simulink model "bus_roadtest_v3"  (R2018a)
settings: Solver=ode3  StartTime=0.0  StopTime=inf  FixedStep=0.01  RelTol=1e-3  EnableMultiTasking=on
PostLoadFcn:
  | , if any(exist('dsrtsu_mdlpostloadfcn', 'file') == [2, 3, 6]), try dsrtsu_mdlpostloadfcn('Execute', bdroot); catch fprintf('Error in PostLoadFcn (dsrtsu_mdlpostloadfcn) for model "%s":\n %s\n', bdroot, lasterr); end, end,
InitFcn:
  | bus_roadtest_v3_initial
values from neighbouring files (symbols this model uses):
  ay_max = 2    [Ini.m]
  delta_t = 0.01    [Ini.m]
  end_left_pass = 1    [Ini.m]
  end_right_pass = 0    [Ini.m]
  finish_node_id = length(Map_data(:,1))    [Ini.m]
  forward_length = 15    [Ini.m]
  gamma = sqrt(N_xaug+lambda)    [bus_roadtest_v3_initial.m]
  k_safe = 1    [Ini.m]
  nodes = nodes(1:index_node,:)    [Ini.m]
  rmin = 10    [Ini.m]
  segments = zeros(length(xy_ends_Pos(:,1)),3)    [Ini.m]
  start_node_id = 1    [Ini.m]
  Ts = 0.01    [bus_roadtest_v3_initial.m]
  Veh_CG = [0.5, 0.2]    [Ini.m]
  Veh_size = [1.99986,6.09558]    [Ini.m]
  vmax = 6    [Ini.m]
  weight = [weight_0,weight_0_cov,weight_i]    [bus_roadtest_v3_initial.m]
undefined symbols (not defined in the file or in its folder): Brake_table, DiscIntNeverNeededParam, Map_data, R, REF_GPS_RFS, Steer_gain_table, T
libraries: rtican x71, simulink x26, rti1401lib_adc_type4 x8, rti1401lib_dio_type4 x1
(part 1 of 18)
settings Model: DSRTSU_INTERNAL_RTI_VER=520  DSRTSU_INTERNAL_RTI_TYPE=rti1401  DSRTSU_INTERNAL_RTIFPGA=110  RTICANMMDATA=struct('GeneralSetupData',struct('modelroot','C:\Users\ITRI\Desktop\CarB_v3','generalsettings',struct('filesettings',struct('destfolder',struct('Name','RTICANMM_FILES','Check',1),'buildfolder',struct('Name','.','Check',1),'AbsDestfolder',struct('Name','C:\Users\ITRI\Desktop\CarB_v3\RTICANMM_FILES'),'AbsBuildfolder',struct('Name','C:\Users\ITRI\Desktop\CarB_v3'))),'options',struct('addpaths',1,'rmpaths',1,'addtrcexclusion',logical(1),'cannavigator',struct('checkmonitoring',0),'show_usrtrc',0,'use_usrtrc',0),'advanced',struct('options',[1 1 1 1 1 1 1 1 1 1 1 1 1 1 1 1 1 1 1 1 1 1 1 1 1 1 1 1 1 1 1 1 1 1 1 1 1 1 1 1 1 1 1 1 1 1 1 1 1 1 1 1 1 1 1 1 1 1 1 1 1 1 1 1 1 1 1 1 1 1 1 1 1 1 1 1 1 1 1 1 1 1 1 1 1 1 1 1 1 1 1 1 1 1 1 1 1 1 1 1]),'MPSetup',{{}},'modelname','bus_roadtest_v3','block','bus_roadtest_v3'))  DSRTSU_INTERNAL_RTIFLEXRAYCONFIG=110  Creator=LABTEST  LastModifiedBy=ITRI
settings DataIOCC: LimitDataPoints=on  SaveFormat=Array
settings OptimizationCC: BlockReduction=off  OptimizeBlockIOStorage=off  BufferReuse=off  GlobalBufferReuse=off  ExpressionFolding=off  ExpressionDepthLimit=2147483647  LocalBlockOutputs=off  LifeSpan=inf  OptimizeDataStoreBuffers=off  BusAssignmentInplaceUpdate=off
settings DebuggingCC: UnderspecifiedInitializationDetection=Classic  MergeDetectMultiDrivingBlocksExec=none  SolverPrmCheckMsg=warning  StateNameClashWarn=warning  SFUnexpectedBacktrackingDiag=warning  SFNoUnconditionalDefaultTransitionDiag=warning  SFExecutionAtInitializationDiag=none
settings HardwareCC: ProdBitPerPointer=32  ProdBitPerSizeT=32  ProdBitPerPtrDiffT=32  ProdLargestAtomicInteger=Integer  ProdEndianess=BigEndian  ProdWordSize=32  ProdHWDeviceType=Custom Processor->Custom  TargetIntDivRoundTo=Zero  TargetEndianess=BigEndian  TargetHWDeviceType=Custom Processor->Custom
settings ModelReferenceCC: PropagateSignalLabelsOutOfModel=off
settings SFSimCC: MATLABDynamicMemAlloc=off
settings RTWCC: SystemTargetFile=rti1401.tlc  MakeCommand=make_rti  TemplateMakefile=rti1401.tmf  Description=dSPACE DS1401 Hardware Platform
settings CodeAppCC: StateflowObjectComments=on
settings STFCustomTargetCC: ParMdlRefBuildCompliant=on  GRTInterface=off  SystemTargetFile=rti1401.tlc
settings GRTTargetCC: TargetLangStandard=C89/C90 (ANSI)  CompOptLevelCompliant=off  ConcurrentExecutionCompliant=off  CombineOutputUpdateFcns=off  MatFileLogging=off  CPPClassGenCompliant=off  UseToolchainInfoCompliant=off  ExtModeMexFile=noextcomm
settings ConfigComp: CovMetricSettings=dw  CovHtmlReporting=on  CovSaveCumulativeToWorkspaceVar=on  CovSaveSingleToWorkspaceVar=on  CovExternalEMLEnable=off
settings SimscapeCC: SimscapeNormalizeSystem=off
settings ConfigurationSet: Description=SimMechanics 2G

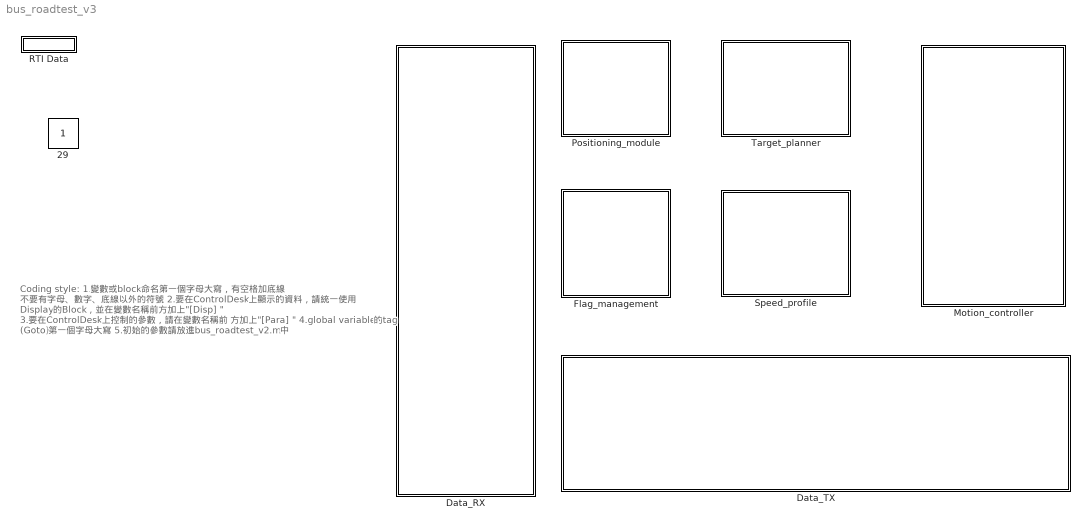
== system bus_roadtest_v3 ==
  note: Coding style:
      | 1.變數或block命名第一個字母大寫，有空格加底線
      | 不要有字母、數字、底線以外的符號
      | 2.要在ControlDesk上顯示的資料，請統一使用
      | Display的Block，並在變數名稱前方加上"[Disp] "
      | 3.要在ControlDesk上控制的參數，請在變數名稱前
      | 方加上"[Para] "
      | 4.global variable的tag (Goto)第一個字母大寫
      | 5.初始的參數請放進bus_roadtest_v2.m中
  Data_RX : Subsystem
  Data_TX : Subsystem
  Flag_management : Subsystem
  Motion_controller : Subsystem
  Positioning_module : Subsystem
  RTI Data : Subsystem  Tag=struct('RTIDataServer',struct('RTIDataServerVs','2','RTIModelDescription','struct(''main'',''bus_roadtest_v3'',''sub'','''',''isMp'',0)'))  LoadFcn="if exist('rtidc'), try,  rtidc('DataHostBlockClbLoad', gcbh); catch, disp(['Warning: ''LoadFcn'' for RTI Data block failed: ' lasterr]); end, end,"  mask(RTI_DATA_HOST){}
      mask help:
      | RTI Data Block.
      | This block is used by RTI to store internal model-dependent data.
      | Please keep this block on the root level of the model. Deleting this block will result in data loss.
      |
      | NEVER DELETE OR COPY THIS BLOCK!
      settings: CopyFcn="if exist('rtidc'), try,  rtidc('DataHostBlockClbCopy', gcbh); catch, disp(['Warning: ''CopyFcn'' for RTI Data block failed: ' lasterr]); end, end,"  DeleteFcn="if exist('rtidc'), try,  rtidc('DataHostBlockClbDelete', gcbh); catch, disp(['Warning: ''DeleteFcn'' for RTI Data block failed: ' lasterr]); end, end,"  ModelCloseFcn="if exist('rtidc'), try,  rtidc('DataHostBlockClbModelClose', gcbh); catch, disp(['Warning: ''ModelCloseFcn'' for RTI Data block failed: ' lasterr]); end, end,"  PreSaveFcn="if exist('rtidc'), try,  rtidc('DataHostBlockClbPreSave', gcbh); catch, disp(['Warning: ''PreSaveFcn'' for RTI Data block failed: ' lasterr]); end, end,"  PostSaveFcn="if exist('rtidc'), try,  rtidc('DataHostBlockClbPostSave', gcbh); catch, disp(['Warning: ''PostSaveFcn'' for RTI Data block failed: ' lasterr]); end, end,"  NameChangeFcn="if exist('rtidc'), try,  rtidc('DataHostBlockClbNameChange', gcbh); catch, disp(['Warning: ''NameChangeFcn'' for RTI Data block failed: ' lasterr]); end, end,"
      mask Help:
      | RTI Data Block.
      | This block is used by RTI to store internal model-dependent data.
      | Please keep this block on the root level of the model. Deleting this block will result in data loss.
      | 
      | NEVER DELETE OR COPY THIS BLOCK!
      mask Display:
      | text(0.5, 0.5, 'RTI Data', 'HorizontalAlignment', 'center');
      | plot([1 0]);
  Speed_profile : Subsystem
  Target_planner : Subsystem
  29 : Constant  IOType=siggen

== system bus_roadtest_v3/Data_RX ==
  note: 請把處理完的資料放在各自的Block裡面
      | 用global variable傳
  Control_button : Subsystem
  OBU : Subsystem
  PLC : Subsystem
  SBG : Subsystem
  X-by-wire : Subsystem
  Xavier : Subsystem

== system bus_roadtest_v3/Data_TX ==
  ARTC : Subsystem
  IPC : Subsystem

== system bus_roadtest_v3/Flag_management ==
  AEB_Enable : Constant
  AEB_Set : Constant  Value=0
  Button management : Subsystem
  Fault detection : Subsystem
  MATLAB Function : MATLAB Function  TreatAsAtomicUnit=on
  Memory : Memory
  Multiport Switch : MultiPortSwitch  DataPortOrder=Specify indices
  Multiport Switch1 : MultiPortSwitch  DataPortOrder=Specify indices
  OR : Logic  Operator=OR  IconShape=distinctive  AllPortsSameDT=off  OutDataTypeStr=boolean
  OR1 : Logic  Operator=OR  IconShape=distinctive  AllPortsSameDT=off  OutDataTypeStr=boolean
  Slow_flag : Constant  Value=0
  State management : Subsystem
  State toggle : MATLAB Function  TreatAsAtomicUnit=on
  "[Disp] AEB_flag_final" : Scope
  "[Disp] Drive_start" : Display
  "[Disp] Drive_state" : Display
  "[Disp] Drive_stop" : Display
  "[Disp] Self_driving_on" : Display
  "[Para] Button_on" : Constant
  "[Para] Door_cmd" : Constant  Value=0
  "[Para] Drive_start" : Constant  Value=0
  "[Para] Drive_stop" : Constant  Value=0
  "[Para] Emergency_stop" : Constant  Value=0
  "[Para] Fault_minor" : Constant  Value=0
  "[Para] Fault_prime" : Constant  Value=0
  switch : Switch  Criteria=u2 > Threshold
  tag scope: AEB_flag=global, BusStop_flag=global, Door_cmd=global, Drive_start=global, Drive_stop=global, Emergency_stop=global, Fault_minor=global, Fault_prime=global, Idle_flag=global, Light_flag=global, Obj_detect=global, Self_driving_on=global, Slow_flag=global, Stop_Check=global, Uturn_flag=global
  wires:
  State management/1(Idle_flag) -> [Idle_flag]
  State management/6(Obj_detect) -> [Obj_detect]
  State management/5(Stop_Check) -> [Stop_Check]
  State management/7(Light_flag) -> [Light_flag]
  State management/8(BusStop_flag) -> [BusStop_flag]
  "[Para] Door_cmd"/1 -> [Door_cmd]
  "[Para] Emergency_stop"/1 -> [Emergency_stop]
  switch/1 -> "[Disp] AEB_flag_final"/1, [AEB_flag]
  AEB_Enable/1 -> switch/2
  AEB_Set/1 -> switch/3
  State management/3(AEB_flag) -> switch/1
  Slow_flag/1 -> [Slow_flag]
  "[Para] Fault_minor"/1 -> [Fault_minor]
  "[Para] Fault_prime"/1 -> [Fault_prime]
  Multiport Switch/1 -> "[Disp] Drive_start"/1, [Drive_start], State toggle/1(Drive_start)
  "[Para] Drive_stop"/1 -> Multiport Switch1/2
  Multiport Switch1/1 -> "[Disp] Drive_stop"/1, State toggle/2(Drive_stop), [Drive_stop]
  "[Para] Button_on"/1 -> Multiport Switch/1, Multiport Switch1/1
  State management/4(Uturn_flag) -> [Uturn_flag]
  [Static_flag] -> State toggle/3(Static_flag)
  State toggle/1(Self_driving_on) -> Memory/1, "[Disp] Self_driving_on"/1, [Self_driving_on]
  "[Para] Drive_start"/1 -> Multiport Switch/2
  [TouchP_start] -> MATLAB Function/3(TouchP_start)
  MATLAB Function/1(Drive_start) -> OR/2
  [Drive_start_button] -> OR/1, Multiport Switch/3
  [Drive_stop_button] -> OR1/2, Multiport Switch1/3
  MATLAB Function/2(Drive_stop) -> OR1/1
  OR1/1 -> Multiport Switch1/4
  OR/1 -> Multiport Switch/4
  [System_ready] -> MATLAB Function/5(System_ready)
  Memory/1 -> MATLAB Function/6(Actual_state)
  [AEB_flag] -> State toggle/4(AEB_flag)
  [TouchP_start_RX] -> MATLAB Function/4(TouchP_start_RX)
  [Drive_start_button] -> MATLAB Function/1(Drive_start_button)
  [Drive_stop_button] -> MATLAB Function/2(Drive_stop_button)
  MATLAB Function/3(Drive_state_out) -> "[Disp] Drive_state"/1
  [Idle_flag] -> State toggle/5(Idle_flag)

== system bus_roadtest_v3/Motion_controller ==
  Auto_flag : Constant
  Constant : Constant  Value=0
  Lateral_control : Subsystem
  Longitudinal_control : Subsystem
  Speed_cmd : Constant  Value=0
  Switch : Switch  Criteria=u2 > Threshold
  Switch1 : Switch  Criteria=u2 > Threshold
  Switch2 : Switch  Criteria=u2 > Threshold
  "[Disp] Speed_cmd" : Display
  "[Para]Speed_cmd_switch" : Constant  Value=0
  wires:
  Switch/1 -> Longitudinal_control/1(Speed_profile), "[Disp] Speed_cmd"/1
  "[Para]Speed_cmd_switch"/1 -> Switch/2
  [Speed_cmd] -> Switch/1
  Speed_cmd/1 -> Switch/3
  Switch1/1 -> Longitudinal_control/2(AEB_trig)
  [AEB_flag] -> Switch1/1
  Constant/1 -> Switch2/3, Switch1/3
  Switch2/1 -> Longitudinal_control/3(Static)
  [Static_flag] -> Switch2/1
  Auto_flag/1 -> Switch2/2, Switch1/2

== system bus_roadtest_v3/Positioning_module ==
  note: 綠底部分為從感測器進來的資訊
  Constant2 : Constant  Value=REF_GPS_RFS
  Gain : Gain  Gain=pi/180
  ITRI_MM : Subsystem
  "[Disp] Sensor_Velocity" : Display
  "[Para] D_GC" : Constant  Value=3.8
  wires:
  [MB5000_Latitude] -> ITRI_MM/2(GPS_LAT)
  [MB5000_Longitude] -> ITRI_MM/1(GPS_LONG)
  [MB5000_Altitude] -> ITRI_MM/3(GPS_ALT)
  [SBG_Course] -> ITRI_MM/6(course)
  Constant2/1 -> ITRI_MM/7(REF_GPS_RFS)
  [SBG_GPS_TYPE] -> ITRI_MM/8(SBG_GPS_TYPE)
  [MB5000_X_Acc] -> ITRI_MM/9(GPS_X_ACC)
  [MB5000_Y_Acc] -> ITRI_MM/10(GPS_Y_ACC)
  [SBG_Longitude] -> ITRI_MM/11(SBG_long)
  [SBG_Latitude] -> ITRI_MM/12(SBG_lat)
  [SBG_Altitude] -> ITRI_MM/13(SBG_alt)
  [SBG_Yaw] -> ITRI_MM/14(SBG_Yaw)
  "[Para] D_GC"/1 -> ITRI_MM/15(D_GC)
  [SLAM_x] -> ITRI_MM/16(SLAM_X)
  [SLAM_y] -> ITRI_MM/17(SLAM_Y)
  [SLAM_heading] -> ITRI_MM/18(SLAM_Heading)
  [SLAM_counter] -> ITRI_MM/19(SLAM_Counter)
  [SLAM_fs] -> ITRI_MM/20(SLAM_FS)
  [SLAM_fault] -> ITRI_MM/21(SLAM_fault)
  [Speed_mps] -> "[Disp] Sensor_Velocity"/1, ITRI_MM/5(Car_Velocity)
  [angular_vz] -> Gain/1
  Gain/1 -> ITRI_MM/4(Car_Yaw_Rate)

== system bus_roadtest_v3/RTI Data ==
  RTI Data Store : Subsystem  Tag="struct('public',struct('sub',struct('name',{{'bus_roadtest_v3'}},'data',{{struct('TH',struct('thTaskInfo',struct('taskType',{'TIMER','HWINT','TMRINT','SWINT','GLINT'},'tasksNumOf',{1,0,0,0,0},'srcIds',{{'TIMERA'},{},{},{},{}},'taskNames',{{['Timer Task 1']},{},{},{},{}})),'th_tc',struct('dataType','TASK','taskGroupId','','taskGroupList',{{}},'taskSchedulingPolicy','FCFS','taskType','TIMER','blkh',-1,'srcId','TIMERA','srcSgnName',['Timer A interrupt'],'srcCpuName','','taskName',['Timer Task 1  [0.01] s'],'taskNameDisplayExt','','smplTime',0.01,'smplTimeOffs',0,'hasFixedPriority',0,'priority',1,'hasFixedOvc',0,'ovcType',1,'ovcMax',1),'tc_th',struct('dataType','TASK','taskGroupId','','taskGroupList',{{}},'taskSchedulingPolicy','FCFS','taskType','TIMER','blkh',-1,'srcId','TIMERA','srcSgnName',['Timer A interrupt'],'srcCpuName','','taskName',['Timer Task 1  [0.01] s'],'taskNameDisplayExt','','smplTime',0.01,'smplTimeOffs',0,'hasFixedPriority',0,'priority',1,'hasFixedOvc',0,'ovcType',1,'ovcMax',1))}})),'private',struct('version',struct('dsVer',uint32(2)),'access',struct('modified',['08-Apr-2020 10:52:29'],'type','Model','isPerm',1)))"  mask(RTI_DATA_STORE){}
      mask help:
      | RTI Data Store Block. This block is used by RTI to store internal model dependent data. Deleting this block will result in data loss.
      |
      | NEVER DELETE, COPY, OR MODIFY THIS BLOCK!
      mask Help:
      | RTI Data Store Block. This block is used by RTI to store internal model dependent data. Deleting this block will result in data loss.
      | 
      | NEVER DELETE, COPY, OR MODIFY THIS BLOCK!
      mask Display: text(0.5, 0.5, ' ', 'HorizontalAlignment', 'center');

== system bus_roadtest_v3/Speed_profile ==
  Auto & Check : Subsystem
  Constant : Constant  Value=0
  Constant1 : Constant  Value=0
  High level controller : Subsystem
  "[Para] Static_flag" : Constant  Value=0
  tag scope: Auto_Door=global, Auto_Start=global, Speed_cmd=global, Static_flag=global
  wires:
  Constant/1 -> [Auto_Door]
  Constant1/1 -> [Auto_Start]
  Auto & Check/1(Static_flag) -> [Static_flag]
  High level controller/1(Speed_cmd) -> [Speed_cmd]

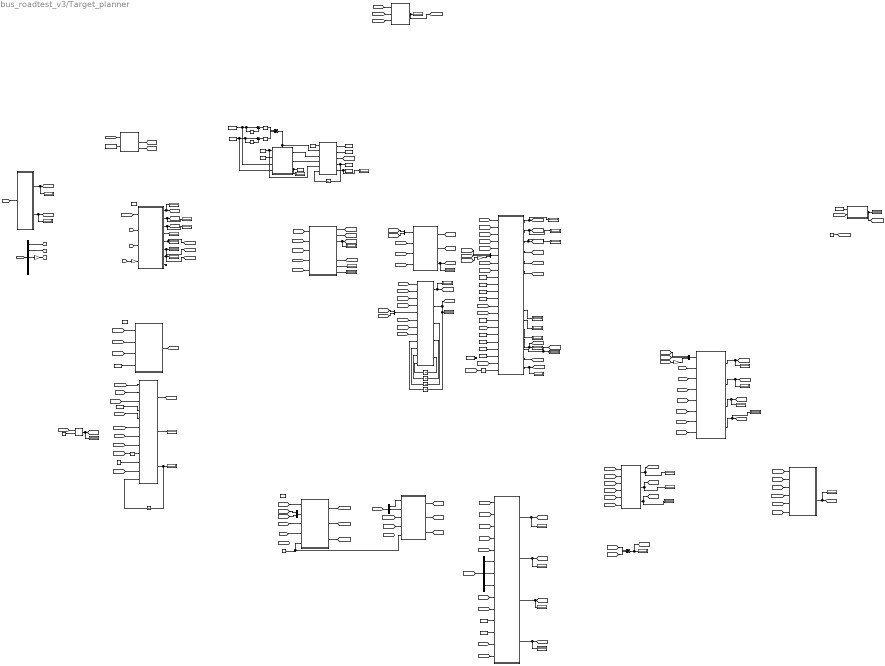
== system bus_roadtest_v3/Target_planner ==
  note: Dynamic Path_1 模組
  note: Dynamic Path_2 模組
  Abs : Abs
  Abs1 : Abs
  Add : Sum
  Add1 : Sum
  Boundingbox_trans : MATLAB Function  TreatAsAtomicUnit=on
  Constant : Constant
  Constant{1..2,6,17,22} (5 alike) : Constant  Value=Map_data
  Constant10 : Constant  Value=end_right_pass
  Constant11 : Constant  Value=end_left_pass
  Constant12 : Constant  Value=Veh_CG
  Constant13 : Constant  Value=Veh_size
  Constant14 : Constant  Value=Veh_size
  Constant15 : Constant  Value=forward_length
  Constant16 : Constant  Value=rmin
  Constant18 : Constant  Value=delta_t
  Constant19 : Constant  Value=ay_max
  Constant20 : Constant  Value=vmax
  Constant21 : Constant  Value=k_safe
  Constant27 : Constant  Value=10
  Constant3 : Constant  Value=nodes
  Constant4 : Constant  Value=Veh_CG
  Constant5 : Constant  Value=segments
  Constant7 : Constant  Value=start_node_id
  Constant8 : Constant  Value=finish_node_id
  Constant9 : Constant  Value=forward_length
  DangerousArea : MATLAB Function  TreatAsAtomicUnit=on  SystemSampleTime=0.01
  Demux : Demux  Outputs=5
  Demux1 : Demux  Outputs=3
  Demux2 : Demux  Outputs=3
  DynamicPathPlanning : MATLAB Function  TreatAsAtomicUnit=on  SystemSampleTime=0.01
  DynamicPathPlanning1 : MATLAB Function  TreatAsAtomicUnit=on  SystemSampleTime=0.01
  Enabled Subsystem : Subsystem  TreatAsAtomicUnit=on
  EndPointDecision : MATLAB Function  TreatAsAtomicUnit=on  SystemSampleTime=0.01
  EndPointDecision1 : MATLAB Function  TreatAsAtomicUnit=on  SystemSampleTime=0.01
  Final_Static_Path : MATLAB Function  TreatAsAtomicUnit=on  SystemSampleTime=0.01
  Forward_Length_Decision : MATLAB Function  TreatAsAtomicUnit=on
  Forward_Seg : MATLAB Function  TreatAsAtomicUnit=on  SystemSampleTime=0.01
  Forward_Seg1 : MATLAB Function  TreatAsAtomicUnit=on  SystemSampleTime=0.01
  Forward_Seg_0 : MATLAB Function  TreatAsAtomicUnit=on
  Gain : Gain  Gain=pi/180
  Gain1 : Gain  Gain=pi/180
  Gain2 : Gain  Gain=pi/180
  Gain3 : Gain  Gain=180/pi
  MATLAB Function : MATLAB Function  TreatAsAtomicUnit=on
  MATLAB Function1 : MATLAB Function  TreatAsAtomicUnit=on
  MM : MATLAB Function  TreatAsAtomicUnit=on  SystemSampleTime=0.01
  Memory : Memory
  Memory1 : Memory
  Mux : Mux  Inputs=2
  Mux1 : Mux  Inputs=2
  Mux2 : Mux  Inputs=3
  Mux3 : Mux  Inputs=2
  Mux4 : Mux  Inputs=3
  Path_Output : MATLAB Function  TreatAsAtomicUnit=on
  Steer_gain_scheduling : MATLAB Function  TreatAsAtomicUnit=on
  Sum : Sum  Inputs=|+-
  Sum1 : Sum  Inputs=|+-
  Target_Point_seg_info1 : MATLAB Function  TreatAsAtomicUnit=on
  Terminator_1 : Terminator
  Terminator_3 : Terminator
  To Workspace1 : ToWorkspace  VariableName=path  SaveFormat=Structure  SampleTime=-1
  To Workspace2 : ToWorkspace  VariableName=dist  SampleTime=-1
  To Workspace3 : ToWorkspace  VariableName=Static_Path_x  SaveFormat=Structure  SampleTime=-1
  To Workspace4 : ToWorkspace  VariableName=Static_Path_y  SaveFormat=Structure  SampleTime=-1
  To Workspace5 : ToWorkspace  VariableName=path_index  SampleTime=-1
  Unit Delay{,1..2,8,12} (5 alike) : UnitDelay  SampleTime=-1
  Unit Delay10 : UnitDelay  InitialCondition=[0 0 0 0]  SampleTime=-1
  Unit Delay5 : UnitDelay  InitialCondition=zeros(11,2)  SampleTime=-1
  Unit Delay9 : UnitDelay  InitialCondition=[0 0 0 0]  SampleTime=-1
  "[Disp] Forward_Static_Path_id" : Display
  "[Disp] J" : Display
  "[Disp] J_finalind" : Display
  "[Disp] Jminind" : Display
  "[Disp] OB_num" : Display
  "[Disp] Path_LV" : Display
  "[Disp] Path_final" : Display
  "[Disp] Path_final_1" : Display
  "[Disp] Path_final_2" : Display
  "[Disp] Path_flag" : Display
  "[Disp] TargetXY" : Display
  "[Disp] Target_seg_heading" : Display
  "[Disp] V_boundingbox" : Display
  "[Disp] Vehicle_Target_x" : Display
  "[Disp] Vehicle_Target_y" : Display
  "[Disp] XP_final" : Display
  "[Disp] XP_final_1" : Display
  "[Disp] XP_final_2" : Display
  "[Disp] YP_final" : Display
  "[Disp] YP_final_1" : Display
  "[Disp] YP_final_2" : Display
  "[Disp] avoidancemode" : Display
  "[Disp] case_0" : Display
  "[Disp] collision_check" : Display
  "[Disp] collision_check_1" : Display
  "[Disp] collision_check_2" : Display
  "[Disp] diffheading" : Display
  "[Disp] end_ind" : Display
  "[Disp] forward_check" : Display
  "[Disp] num_lane_direction" : Display
  "[Disp] oi_near" : Display
  "[Disp] op_dist" : Display
  "[Disp] path" : Display
  "[Disp] path_index" : Display
  "[Disp] path_length" : Display
  "[Disp] seg_Curvature" : Display
  "[Disp] seg_LaneWidth" : Display
  "[Disp] seg_heading" : Display
  "[Disp] seg_id_near" : Display
  "[Disp] target_seg_id" : Display
  "[Disp] vehicle_boundingbox_x" : Display
  "[Disp] vehicle_boundingbox_y" : Display
  "[Disp] vehicle_position" : Display
  "[Disp] w_off" : Display
  "[Para] Override_length" : Constant  Value=15
  "[Para] Path_flag_switch" : Constant  Value=0
  "[Para] Steer_gain_table" : Constant  Value=Steer_gain_table
  "[Para] forward_length_2" : Constant  Value=15
  target_seg_id_search : MATLAB Function  TreatAsAtomicUnit=on  SystemSampleTime=0.01
  trajectory merge : MATLAB Function  TreatAsAtomicUnit=on
  tag scope: End_x=global, End_x_1=global, End_y=global, End_y_1=global, Forward_Static_Path_id=global, Forward_Static_Path_id_1=global, Forward_Static_Path_x=global, Forward_Static_Path_x_1=global, Forward_Static_Path_y=global, Forward_Static_Path_y_1=global, J_finalind=global, Jminind=global, K_gain=global, L_path_final=global, Look_ahead_S0=global, OB_num=global, Oi_near=global, Path_LV=global, Path_final=global, Path_final_1=global, Path_final_2=global, Rotz=global, Static_Path_0=global, TargetXY=global, Target_seg_heading=global, Target_seg_id=global, V_boundingbox=global, Vehicle_Target_x=global, Vehicle_Target_y=global, X=global, XP_final=global, XP_final_1=global, XP_final_2=global, Y=global, YP_final=global, YP_final_1=global, YP_final_2=global, avoidancemode=global, collision_check=global, collision_check_1=global, collision_check_2=global, end_curvature=global, end_point_final=global, end_seg_id=global, forward_length=global, op_dist=global, path_length=global, path_length_1=global, seg_Curvature=global, seg_LaneWidth=global, seg_heading=global, seg_id_near=global, target_seg_id=global, v_final=global, vehicle_position=global, w_off=global
  wires:
  Memory1/1 -> Sum1/2
  "[Para] forward_length_2"/1 -> EndPointDecision1/5(forward_length), Forward_Seg1/5(forward_length)
  EndPointDecision/3(path_length) -> "[Disp] path_length"/1, [path_length]
  DynamicPathPlanning/10(vehicle_boundingbox_x) -> "[Disp] vehicle_boundingbox_x"/1
  Gain3/1 -> [Rotz]
  MM/1(seg_id_near) -> [seg_id_near], "[Disp] seg_id_near"/1
  Constant11/1 -> DynamicPathPlanning/10(end_left_pass)
  Demux/3 -> Gain3/1
  Demux/1 -> [X]
  Forward_Seg1/3(Forward_Static_Path_id) -> [Forward_Static_Path_id_1]
  [X] -> MM/2(Position_X)
  [collision_check_1] -> Add1/2
  Constant2/1 -> Target_Point_seg_info1/1(Map_data)
  Unit Delay9/1 -> DangerousArea/10(last_H_x)
  Constant7/1 -> Enabled Subsystem/3(start_id), Memory1/1, Sum1/1
  Sum1/1 -> Abs1/1
  MM/5(seg_heading) -> "[Disp] seg_heading"/1, [seg_heading]
  MATLAB Function/4(TargetXY) -> "[Disp] TargetXY"/1, [TargetXY]
  MM/2(op_distance) -> "[Disp] op_dist"/1, [op_dist]
  DynamicPathPlanning/4(v_final) -> [v_final]
  DangerousArea/5(count_o) -> Unit Delay12/1
  [Static_Path_0] -> MM/1(Map_data)
  [V_boundingbox] -> DangerousArea/2(OBXY)
  Constant/1 -> [Target_seg_id]
  [U_turn] -> Steer_gain_scheduling/1(U_turn)
  Boundingbox_trans/2(V_boundingbox) -> "[Disp] V_boundingbox"/1, [V_boundingbox]
  [Target_seg_id] -> Target_Point_seg_info1/2(Target_seg_id)
  Steer_gain_scheduling/2(Look_ahead_S0) -> [Look_ahead_S0]
  [avoidancemode] -> Unit Delay1/1
  "[Para] Steer_gain_table"/1 -> Steer_gain_scheduling/2(Steer_gain_table)
  Boundingbox_trans/1(OB_num) -> "[Disp] OB_num"/1, [OB_num]
  MM/7(seg_Curvature) -> [seg_Curvature], "[Disp] seg_Curvature"/1
  Final_Static_Path/2(Static_Path_y) -> To Workspace4/1
  [X_UKF_SLAM] -> Demux/1
  [forwardendheading0] -> Forward_Length_Decision/7(forwardendheading0)
  [Forward_Static_Path_x] -> EndPointDecision/2(Path_x_0)
  [Forward_Static_Path_y] -> EndPointDecision/3(Path_y_0)
  [Speed_mps] -> Forward_Length_Decision/1(Car_velocity)
  DynamicPathPlanning/15(L_path_final) -> [L_path_final]
  Forward_Length_Decision/1(Forward_length_final) -> [forward_length]
  [forward_length] -> Forward_Seg/5(forward_length)
  Abs/1 -> Add/2
  Demux/2 -> [Y]
  [end_curvature] -> DynamicPathPlanning1/9(seg_Curvature)
  [Static_Path_0] -> Forward_Seg_0/1(Static_Path_0)
  [Look_ahead_S0] -> Forward_Length_Decision/2(LAS0)
  Final_Static_Path/4(dist_out) -> Unit Delay/1, To Workspace2/1
  DangerousArea/3(H_x_out) -> Unit Delay9/1
  MM/4(num_lane_direction) -> "[Disp] num_lane_direction"/1
  [Oi_near] -> Forward_Seg_0/2(Vehicle_state)
  Add/1 -> Final_Static_Path/2(onoff), Enabled Subsystem/Enable
  [Static_Path_0] -> Forward_Seg1/1(Static_Path_0)
  Sum/1 -> Abs/1
  [op_dist] -> Forward_Length_Decision/5(op_dist)
  Final_Static_Path/1(Static_Path_x) -> To Workspace3/1
  [OB_num] -> DynamicPathPlanning1/13(OB_num)
  Unit Delay/1 -> Final_Static_Path/6(dist_in)
  [X] -> Mux2/1
  Constant13/1 -> DynamicPathPlanning/12(Veh_size)
  [Y] -> Mux/2
  Unit Delay2/1 -> Forward_Length_Decision/12(forward_check_i)
  [XP_final] -> trajectory merge/1(XP_final)
  [Speed_mps] -> MATLAB Function/2(Veh_Velocity)
  Abs1/1 -> Add/1
  [seg_id_near] -> Forward_Seg_0/3(SEG_ID_NEAR_TRUE)
  [YP_final] -> MATLAB Function/6(YP_final)
  [Path_final] -> trajectory merge/5(Path_final)
  DangerousArea/1(w_off) -> "[Disp] w_off"/1, [w_off]
  [collision_check] -> Add1/1
  EndPointDecision/1(End_x) -> [End_x]
  Steer_gain_scheduling/3(K_gain) -> [K_gain]
  [End_x] -> DynamicPathPlanning/4(End_x)
  [X] -> Mux4/1
  DynamicPathPlanning/3(YP_final) -> "[Disp] YP_final"/1, [YP_final]
  DynamicPathPlanning1/1(Path_final) -> "[Disp] Path_final_1"/1, [Path_final_1]
  Target_Point_seg_info1/1(Target_seg_heading) -> [Target_seg_heading], "[Disp] Target_seg_heading"/1
  [Forward_Static_Path_x] -> Path_Output/2(Path_x)
  [forward_length] -> EndPointDecision/4(forward_length)
  [Y] -> Mux1/2
  Gain1/1 -> Mux2/3
  [Speed_mps] -> Forward_Seg1/4(Car_Velocity)
  Mux4/1 -> MATLAB Function/1(Vehicle_state)
  Enabled Subsystem/3(nn) -> To Workspace5/1, "[Disp] path_index"/1
  [Look_ahead_S0] -> MATLAB Function/3(LAS0)
  EndPointDecision1/1(End_x) -> [End_x_1]
  Constant15/1 -> Forward_Length_Decision/4(Forward_length)
  Mux3/1 -> Forward_Seg1/2(Vehicle_state)
  [Rotz] -> Gain2/1
  [Rotz] -> Gain1/1
  DynamicPathPlanning/16(collision_check) -> "[Disp] collision_check"/1, [collision_check]
  trajectory merge/1(XP_final_2) -> "[Disp] XP_final_2"/1, [XP_final_2]
  Enabled Subsystem/2(path) -> Final_Static_Path/4(path_new)
  Unit Delay5/1 -> DynamicPathPlanning/22(LastPath_in)
  [Y] -> Mux2/2
  Mux1/1 -> DangerousArea/5(vehicle_position)
  DangerousArea/4(H_y_out) -> Unit Delay10/1
  EndPointDecision1/2(End_y) -> [End_y_1]
  Path_Output/1(Path_LV) -> [Path_LV], "[Disp] Path_LV"/1
  DynamicPathPlanning/13(Jminind) -> [Jminind], "[Disp] Jminind"/1
  DynamicPathPlanning/12(J_out) -> "[Disp] J"/1
  [Speed_mps] -> Forward_Seg/4(Car_Velocity)
  DynamicPathPlanning1/3(YP_final) -> "[Disp] YP_final_1"/1, [YP_final_1]
  Constant14/1 -> DynamicPathPlanning1/12(Veh_size)
  [Speed_mps] -> DynamicPathPlanning/16(Veh_Velocity)
  Constant20/1 -> DynamicPathPlanning/19(vmax)
  Unit Delay12/1 -> DangerousArea/12(count_i)
  Constant3/1 -> Final_Static_Path/5(nodes), Enabled Subsystem/1(nodes)
  [End_x_1] -> DynamicPathPlanning1/3(End_x)
  Forward_Seg/6(end_seg_id) -> [end_seg_id]
  [L_path_final] -> MATLAB Function/7(L_path_fianl)
  [Forward_Static_Path_id_1] -> DynamicPathPlanning1/2(Forward_Static_Path_id)
  Gain2/1 -> Mux4/3
  Constant4/1 -> DynamicPathPlanning1/11(Veh_CG)
  trajectory merge/3(Path_final_2) -> "[Disp] Path_final_2"/1, [Path_final_2]
  Final_Static_Path/3(Static_Path_0) -> [Static_Path_0]
  Constant10/1 -> DynamicPathPlanning/9(end_right_pass)
  [Forward_Static_Path_id] -> DangerousArea/6(Forward_Static_Path_id)
  MATLAB Function/3(Vehicle_Target_y) -> "[Disp] Vehicle_Target_y"/1, [Vehicle_Target_y]
  [End_y] -> DangerousArea/4(End_y)
  Constant12/1 -> DynamicPathPlanning/11(Veh_CG)
  [End_y] -> DynamicPathPlanning/5(End_y)
  Forward_Seg/1(Forward_Static_Path_x) -> [Forward_Static_Path_x]
  DangerousArea/2(avoidancemode) -> [avoidancemode], "[Disp] avoidancemode"/1, Unit Delay8/1
  [Rotz] -> Gain/1
  [Static_Path_0] -> DynamicPathPlanning1/1(Static_Path_0)
  Forward_Length_Decision/2(diffheading1) -> "[Disp] diffheading"/1
  [Static_Path_0] -> DangerousArea/7(Static_Path_0)
  [Y] -> MM/3(Postion_Y)
  [End_x] -> DangerousArea/3(End_x)
  [V_boundingbox] -> DynamicPathPlanning1/14(OBXY)
  [End_y] -> Mux3/2
  Forward_Seg/2(Forward_Static_Path_y) -> [Forward_Static_Path_y]
  Unit Delay8/1 -> DangerousArea/9(last_avoidancemode)
  [Y] -> Mux4/2
  [Static_Path_0] -> Forward_Seg/1(Static_Path_0)
  [forward_length] -> DangerousArea/8(forward_length)
  [End_x] -> Mux3/1
  MM/3(Oi_near) -> "[Disp] oi_near"/1, [Oi_near]
  [YP_final] -> trajectory merge/2(YP_final)
  [seg_id_near] -> Forward_Seg/3(SEG_ID_NEAR_TRUE)
  EndPointDecision/2(End_y) -> [End_y]
  Mux2/1 -> DynamicPathPlanning/6(Vehicle_state)
  DynamicPathPlanning/2(XP_final) -> "[Disp] XP_final"/1, [XP_final]
  [Forward_Static_Path_id] -> DynamicPathPlanning/3(Forward_Static_Path_id)
  Forward_Length_Decision/3(forward_check_o) -> Unit Delay2/1, "[Disp] forward_check"/1
  [Forward_Static_Path_x_1] -> EndPointDecision1/3(Path_x_0)
  Mux/1 -> EndPointDecision/1(Vehicle_state)
  [YP_final_1] -> trajectory merge/4(YP_final_1)
  DynamicPathPlanning/6(end_curvature) -> [end_curvature]
  DynamicPathPlanning/5(end_point_final) -> [end_point_final]
  Forward_Seg_0/1(Forward_Static_Path_heading) -> [forwardendheading0]
  Constant6/1 -> Final_Static_Path/1(Map_data)
  DynamicPathPlanning1/2(XP_final) -> "[Disp] XP_final_1"/1, [XP_final_1]
  [Path_final_1] -> trajectory merge/6(Path_final_1)
  [X] -> Mux/1
  [end_seg_id] -> Forward_Seg1/3(SEG_ID_NEAR_TRUE)
  Constant5/1 -> Enabled Subsystem/2(segrments)
  MATLAB Function/1(Vehicle_nextstep) -> "[Disp] vehicle_position"/1, [vehicle_position]
  [Static_Path_0] -> DynamicPathPlanning/2(Static_Path_0)
  Unit Delay10/1 -> DangerousArea/11(last_H_y)
  [Oi_near] -> Forward_Seg/2(Vehicle_state)
  trajectory merge/2(YP_final_2) -> "[Disp] YP_final_2"/1, [YP_final_2]
  DynamicPathPlanning1/4(collision_check) -> "[Disp] collision_check_1"/1, [collision_check_1]
  Enabled Subsystem/1(dist) -> Final_Static_Path/3(dist_new)
  Gain/1 -> MM/4(Position_H)
  Forward_Seg1/1(Forward_Static_Path_x) -> [Forward_Static_Path_x_1]
  Constant9/1 -> Forward_Seg_0/4(forward_length)
  Final_Static_Path/5(path_out) -> "[Disp] path"/1, To Workspace1/1
  [seg_Curvature] -> DynamicPathPlanning/7(seg_Curvature)
  [End_y_1] -> DynamicPathPlanning1/4(End_y)
  Forward_Seg1/2(Forward_Static_Path_y) -> [Forward_Static_Path_y_1]
  Forward_Seg/3(Forward_Static_Path_id) -> "[Disp] Forward_Static_Path_id"/1, [Forward_Static_Path_id]
  Add1/1 -> [collision_check_2], "[Disp] collision_check_2"/1
  Constant16/1 -> DynamicPathPlanning/15(rmin)
  [X] -> Mux1/1
  [XP_final_1] -> trajectory merge/3(XP_final_1)
  [X_UKF_SLAM] -> Path_Output/1(Vehicle_state)
  [OB_num] -> DynamicPathPlanning/13(OB_num)
  Constant19/1 -> DynamicPathPlanning/18(ay_max)
  Unit Delay1/1 -> Forward_Length_Decision/9(avoidancemode)
  DynamicPathPlanning/11(vehicle_boundingbox_y) -> "[Disp] vehicle_boundingbox_y"/1
  [Forward_Static_Path_y_1] -> EndPointDecision1/4(Path_y_0)
  [Forward_Static_Path_y] -> Path_Output/3(Path_y)
  [XP_final] -> MATLAB Function/5(XP_final)
  [Path_final] -> Unit Delay5/1
  [V_boundingbox] -> DynamicPathPlanning/14(OBXY)
  Constant8/1 -> Enabled Subsystem/4(finish_id), Sum/1, Memory/1
  [path_length_1] -> DynamicPathPlanning1/10(path_length)
  [seg_LaneWidth] -> Forward_Length_Decision/6(seg_LaneWidth)
  DynamicPathPlanning/1(Path_final) -> "[Disp] Path_final"/1, [Path_final]
  EndPointDecision1/3(path_length) -> [path_length_1]
  Memory/1 -> Sum/2
  [w_off] -> DynamicPathPlanning/21(w_off)
  MM/6(seg_LaneWidth) -> [seg_LaneWidth], "[Disp] seg_LaneWidth"/1
  [J_finalind] -> DynamicPathPlanning1/5(Jminind)
  [OB_num] -> DangerousArea/1(OB_num)
  Constant18/1 -> DynamicPathPlanning/17(delta_t)
  MATLAB Function/2(Vehicle_Target_x) -> "[Disp] Vehicle_Target_x"/1, [Vehicle_Target_x]
  MM/8(note) -> Terminator_3/1
  Constant27/1 -> Terminator_1/1
  [Rotz] -> Forward_Length_Decision/8(Rotz)
  Constant21/1 -> DynamicPathPlanning/20(k_safe)
  [path_length] -> DynamicPathPlanning/8(path_length)
  [end_point_final] -> Demux1/1
  Demux1/2 -> DynamicPathPlanning1/7(y_vehicle)
  Demux1/3 -> DynamicPathPlanning1/8(start_heading)
  [end_point_final] -> Demux2/1
  Demux2/1 -> EndPointDecision1/1(x)
  Demux2/2 -> EndPointDecision1/2(y)
  Demux1/1 -> DynamicPathPlanning1/6(x_vehicle)
  Forward_Seg/7(case_0) -> "[Disp] case_0"/1
  Forward_Seg/8(end_ind) -> "[Disp] end_ind"/1
  [Path_flag] -> Forward_Length_Decision/11(Path_flag)
  DynamicPathPlanning/14(J_finalind) -> "[Disp] J_finalind"/1, [J_finalind]
  [SLAM_seg_id_near] -> MATLAB Function1/1(ID)
  MATLAB Function1/1(Path_flag) -> "[Disp] Path_flag"/1, [Path_flag]
  [Path_flag] -> DynamicPathPlanning/1(Path_flag)
  "[Para] Override_length"/1 -> Forward_Length_Decision/10(Intrusion_range)
  "[Para] Path_flag_switch"/1 -> MATLAB Function1/2(switch_flag)
  [Path_flag] -> MATLAB Function/8(Detour_flag)
  [X_UKF_SLAM] -> Boundingbox_trans/1(vehicle_state)
  [Ros_Look_ahead_time] -> Forward_Length_Decision/3(LAT)
  [Ros_Look_ahead_time] -> MATLAB Function/4(LAT)
  [Static_Path_0] -> target_seg_id_search/1(Static_Path_0)
  [Speed_mps] -> target_seg_id_search/4(Car_Velocity)
  [Oi_near] -> target_seg_id_search/2(Vehicle_state)
  target_seg_id_search/6(end_seg_id) -> "[Disp] target_seg_id"/1, [target_seg_id]
  [Look_ahead_S0] -> target_seg_id_search/6(LAS0)
  [seg_id_near] -> target_seg_id_search/3(SEG_ID_NEAR_TRUE)
  [Ros_Look_ahead_time] -> target_seg_id_search/5(LAT)
